simulink model "TanksModel"  (R2017b)
settings: Solver=FixedStepAuto  StartTime=0.0  StopTime=300  FixedStep=0.1  RelTol=1e-3
values from neighbouring files (symbols this model uses):
  A1 = 2    [init.m]
  AlarmLevel_NF = 12    [configurationScript.m]
  hmax = 15    [init.m]
  R1 = 5    [init.m]
  R2 = 5    [init.m]
settings Model: Creator=aarrieta  LastModifiedBy=aarrieta

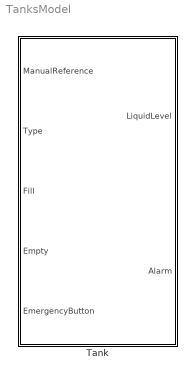
== system TanksModel ==
  Tank : Subsystem

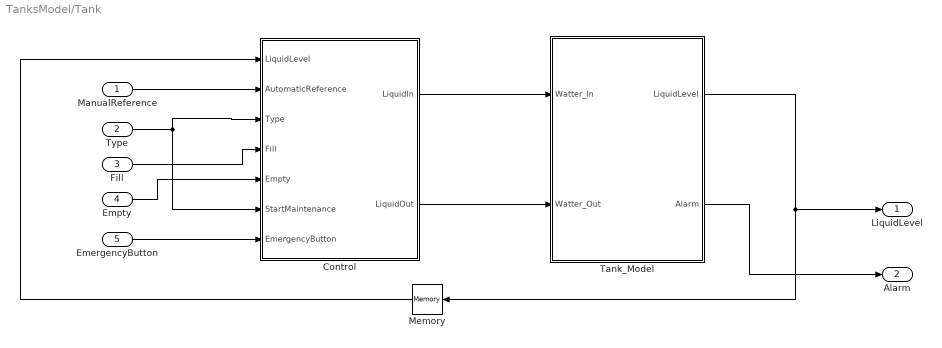
== system TanksModel/Tank ==
  ManualReference : Inport
  Type : Inport  Port=2
  Fill : Inport  Port=3
  Empty : Inport  Port=4
  EmergencyButton : Inport  Port=5
  Control : Subsystem
  Memory : Memory
  Tank_Model : Subsystem
  LiquidLevel : Outport
  Alarm : Outport  Port=2
  wires:
  Tank_Model/1(LiquidLevel) -> Memory/1, LiquidLevel/1
  Control/2(LiquidOut) -> Tank_Model/2(Watter_Out)
  Memory/1 -> Control/1(LiquidLevel)
  ManualReference/1 -> Control/2(AutomaticReference)
  Type/1 -> Control/3(Type), Control/6(StartMaintenance)
  Fill/1 -> Control/4(Fill)
  Empty/1 -> Control/5(Empty)
  EmergencyButton/1 -> Control/7(EmergencyButton)
  Control/1(LiquidIn) -> Tank_Model/1(Watter_In)
  Tank_Model/2(Alarm) -> Alarm/1

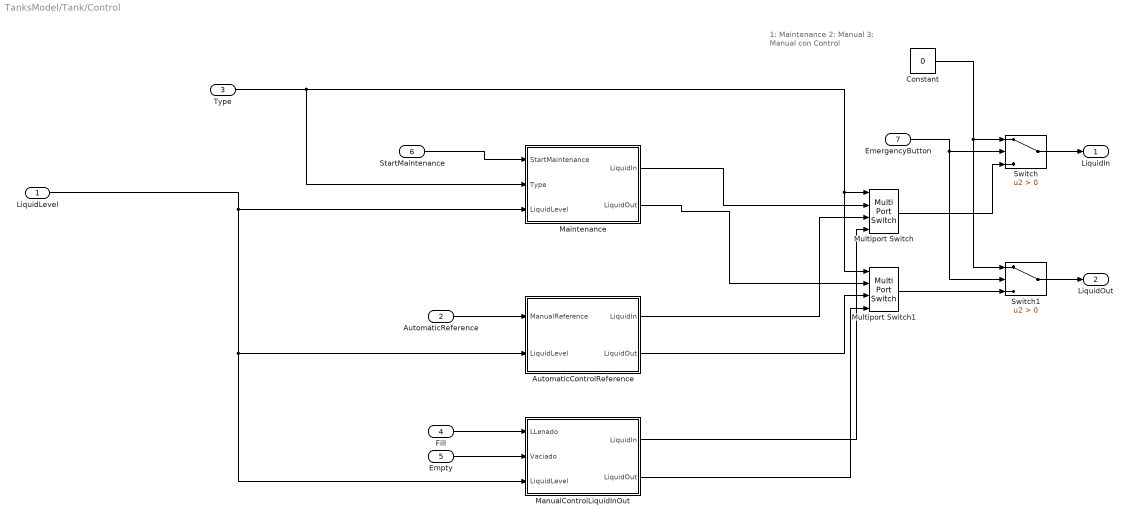
== system TanksModel/Tank/Control ==
  note: 1: Maintenance
      | 2: Manual
      | 3: Manual con Control
  LiquidLevel : Inport
  AutomaticReference : Inport  Port=2
  Type : Inport  Port=3
  Fill : Inport  Port=4
  Empty : Inport  Port=5
  StartMaintenance : Inport  Port=6
  EmergencyButton : Inport  Port=7
  AutomaticControlReference : Subsystem
  Constant : Constant  Value=0
  Maintenance : Subsystem
  ManualControlLiquidInOut : Subsystem
  Multiport Switch : MultiPortSwitch
  Multiport Switch1 : MultiPortSwitch
  Switch : Switch  Criteria=u2 > Threshold
  Switch1 : Switch  Criteria=u2 > Threshold
  LiquidIn : Outport
  LiquidOut : Outport  Port=2
  wires:
  Multiport Switch/1 -> Switch/3
  Multiport Switch1/1 -> Switch1/3
  Type/1 -> Maintenance/2(Type), Multiport Switch1/1, Multiport Switch/1
  Maintenance/1(LiquidIn) -> Multiport Switch/2
  AutomaticControlReference/1(LiquidIn) -> Multiport Switch/3
  Maintenance/2(LiquidOut) -> Multiport Switch1/2
  AutomaticControlReference/2(LiquidOut) -> Multiport Switch1/3
  AutomaticReference/1 -> AutomaticControlReference/1(ManualReference)
  LiquidLevel/1 -> ManualControlLiquidInOut/3(LiquidLevel), AutomaticControlReference/2(LiquidLevel), Maintenance/3(LiquidLevel)
  ManualControlLiquidInOut/1(LiquidIn) -> Multiport Switch/4
  ManualControlLiquidInOut/2(LiquidOut) -> Multiport Switch1/4
  Empty/1 -> ManualControlLiquidInOut/2(Vaciado)
  Fill/1 -> ManualControlLiquidInOut/1(LLenado)
  StartMaintenance/1 -> Maintenance/1(StartMaintenance)
  Switch/1 -> LiquidIn/1
  Switch1/1 -> LiquidOut/1
  Constant/1 -> Switch1/1, Switch/1
  EmergencyButton/1 -> Switch1/2, Switch/2

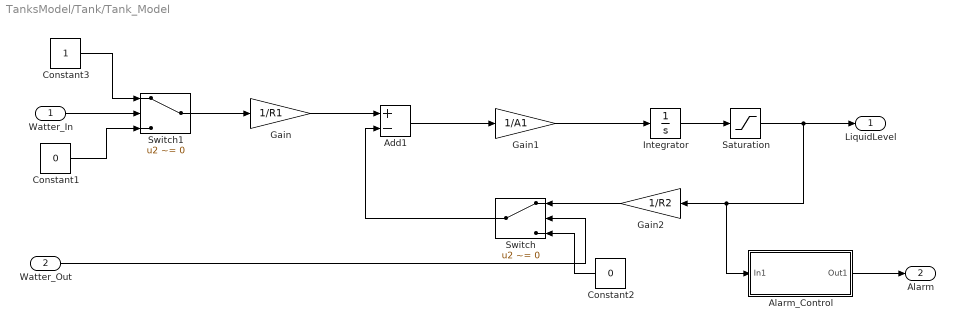
== system TanksModel/Tank/Tank_Model ==
  Watter_In : Inport
  Watter_Out : Inport  Port=2
  Add1 : Sum  Inputs=+-
  Alarm_Control : Subsystem
  Constant1 : Constant  Value=0
  Constant2 : Constant  Value=0
  Constant3 : Constant
  Gain : Gain  Gain=1/R1
  Gain1 : Gain  Gain=1/A1
  Gain2 : Gain  Gain=1/R2
  Integrator : Integrator
  Saturation : Saturate  UpperLimit=hmax  LowerLimit=0
  Switch : Switch  Criteria=u2 ~= 0
  Switch1 : Switch  Criteria=u2 ~= 0
  LiquidLevel : Outport
  Alarm : Outport  Port=2
  wires:
  Watter_Out/1 -> Switch/2
  Add1/1 -> Gain1/1
  Gain2/1 -> Switch/1
  Watter_In/1 -> Switch1/2
  Switch/1 -> Add1/2
  Switch1/1 -> Gain/1
  Constant2/1 -> Switch/3
  Constant3/1 -> Switch1/1
  Integrator/1 -> Saturation/1
  Gain1/1 -> Integrator/1
  Gain/1 -> Add1/1
  Constant1/1 -> Switch1/3
  Alarm_Control/1(Out1) -> Alarm/1
  Saturation/1 -> LiquidLevel/1, Alarm_Control/1(In1), Gain2/1

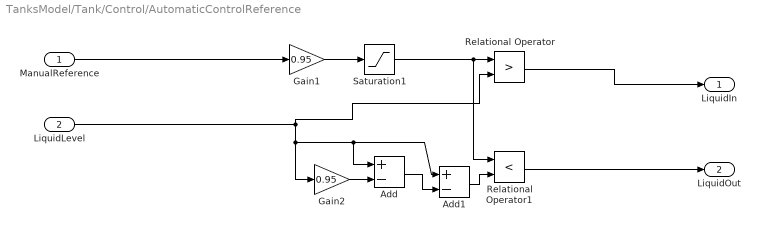
== system TanksModel/Tank/Control/AutomaticControlReference ==
  ManualReference : Inport
  LiquidLevel : Inport  Port=2
  Add : Sum  Inputs=+-
  Add1 : Sum  Inputs=+-
  Gain1 : Gain  Gain=0.95
  Gain2 : Gain  Gain=0.95
  Relational Operator : RelationalOperator  Operator=>  OutDataTypeStr=boolean  RndMeth=Simplest
  Relational Operator1 : RelationalOperator  Operator=<  OutDataTypeStr=boolean  RndMeth=Simplest
  Saturation1 : Saturate  UpperLimit=hmax*0.9  LowerLimit=0
  LiquidIn : Outport
  LiquidOut : Outport  Port=2
  wires:
  LiquidLevel/1 -> Relational Operator/2, Add/1, Add1/1, Gain2/1
  Relational Operator/1 -> LiquidIn/1
  Relational Operator1/1 -> LiquidOut/1
  Add/1 -> Add1/2
  Add1/1 -> Relational Operator1/2
  Gain1/1 -> Saturation1/1
  Gain2/1 -> Add/2
  ManualReference/1 -> Gain1/1
  Saturation1/1 -> Relational Operator1/1, Relational Operator/1

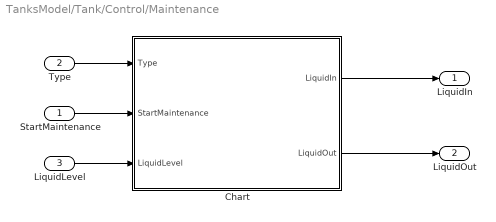
== system TanksModel/Tank/Control/Maintenance ==
  StartMaintenance : Inport
  Type : Inport  Port=2
  LiquidLevel : Inport  Port=3
  Chart : Stateflow chart  TreatAsAtomicUnit=on
  LiquidIn : Outport
  LiquidOut : Outport  Port=2
  wires:
  StartMaintenance/1 -> Chart/2(StartMaintenance)
  Type/1 -> Chart/1(Type)
  LiquidLevel/1 -> Chart/3(LiquidLevel)
  Chart/1(LiquidIn) -> LiquidIn/1
  Chart/2(LiquidOut) -> LiquidOut/1

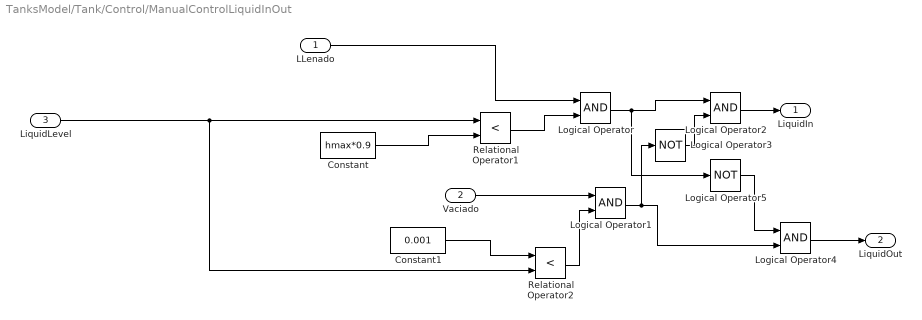
== system TanksModel/Tank/Control/ManualControlLiquidInOut ==
  LLenado : Inport
  Vaciado : Inport  Port=2
  LiquidLevel : Inport  Port=3
  Constant : Constant  Value=hmax*0.9
  Constant1 : Constant  Value=0.001
  Logical Operator{,1..2,4} (4 alike) : Logic  AllPortsSameDT=off  OutDataTypeStr=boolean
  Logical Operator3 : Logic  Operator=NOT  AllPortsSameDT=off  OutDataTypeStr=boolean
  Logical Operator5 : Logic  Operator=NOT  AllPortsSameDT=off  OutDataTypeStr=boolean
  Relational Operator1 : RelationalOperator  Operator=<  OutDataTypeStr=boolean  RndMeth=Simplest
  Relational Operator2 : RelationalOperator  Operator=<  OutDataTypeStr=boolean  RndMeth=Simplest
  LiquidIn : Outport
  LiquidOut : Outport  Port=2
  wires:
  Vaciado/1 -> Logical Operator1/1
  Constant/1 -> Relational Operator1/2
  Relational Operator1/1 -> Logical Operator/2
  LLenado/1 -> Logical Operator/1
  Logical Operator/1 -> Logical Operator5/1, Logical Operator2/1
  Relational Operator2/1 -> Logical Operator1/2
  Logical Operator1/1 -> Logical Operator4/2, Logical Operator3/1
  Constant1/1 -> Relational Operator2/1
  LiquidLevel/1 -> Relational Operator2/2, Relational Operator1/1
  Logical Operator3/1 -> Logical Operator2/2
  Logical Operator2/1 -> LiquidIn/1
  Logical Operator5/1 -> Logical Operator4/1
  Logical Operator4/1 -> LiquidOut/1

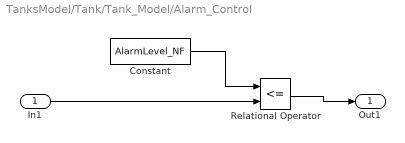
== system TanksModel/Tank/Tank_Model/Alarm_Control ==
  In1 : Inport
  Constant : Constant  Value=AlarmLevel_NF
  Relational Operator : RelationalOperator  Operator=<=  OutDataTypeStr=boolean  RndMeth=Simplest
  Out1 : Outport
  wires:
  In1/1 -> Relational Operator/2
  Constant/1 -> Relational Operator/1
  Relational Operator/1 -> Out1/1

== stateflow chart TanksModel/Tank/Control/Maintenance/Chart ==
  state InitialState
    entry: LiquidIn = 0;
    LiquidOut = 0;
  state Step1
    entry: LiquidIn = 0;
    LiquidOut = 1;
  state Step2
    entry: LiquidIn = 1;
    LiquidOut = 0;
  state Step3
    entry: LiquidIn = 0;
    LiquidOut = 1;
  (default) -> InitialState
  Step3 -> InitialState : [Type~=1||LiquidLevel <=0.01]
  Step2 -> InitialState [order 1] : [Type~=1]
  Step1 -> InitialState [order 1] : [Type ~= 1]
  InitialState -> Step1 : [StartMaintenance == 1 && Type ==1]
  Step1 -> Step2 [order 2] : [LiquidLevel <=0.01]
  Step2 -> Step3 [order 2] : [LiquidLevel>=hmax*0.9]
  data: Type input; StartMaintenance input; LiquidIn output; LiquidOut output; LiquidLevel input; hmax parameter
